simulink model "sim_kalman"  (R2024b)
settings: Solver=ode4  StartTime=t_0  StopTime=t_f  FixedStep=dt  RelTol=1e-8
libraries: simulink x1
settings Model: SimulationMode=accelerator  Creator=yevge  LastModifiedBy=Aiden Gaydos
settings DebuggingCC: AlgebraicLoopMsg=error  CheckMatrixSingularityMsg=error

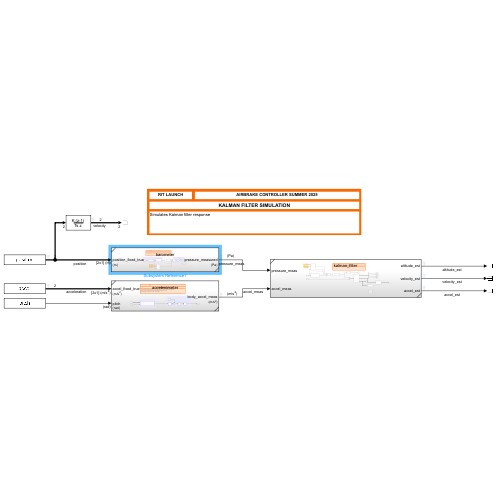
[thumbnail: Simulink's stored preview of the top-level diagram]
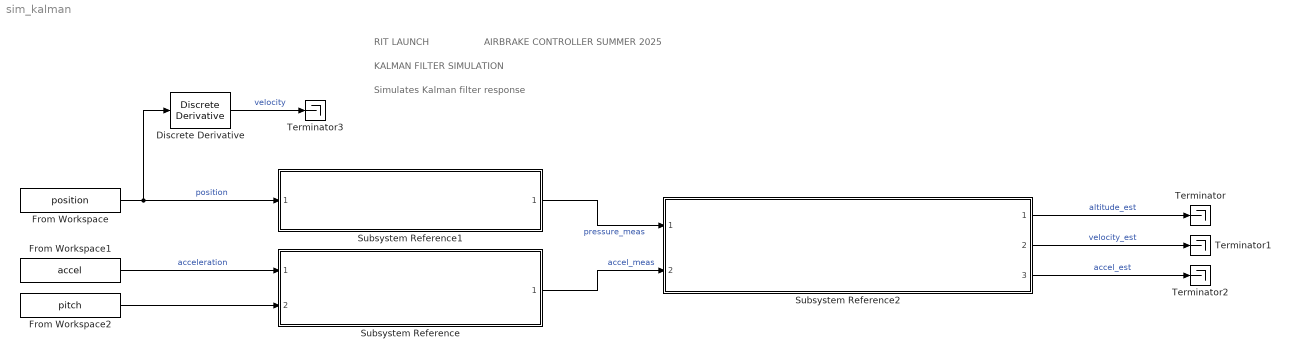
== system sim_kalman ==
  note: AIRBRAKE CONTROLLER SUMMER 2025
  note: RIT LAUNCH
  note: KALMAN FILTER SIMULATION
  note: Simulates Kalman filter response
  Discrete Derivative : simulink/Discrete/Discrete Derivative  gainval=1  ICPrevScaledInput=0.0  OutMin=[]  OutMax=[]  OutDataType=fixdt(1, 16)  OutScaling=2^-10  DoSatur=off
  From Workspace : FromWorkspace  VariableName=position
  From Workspace1 : FromWorkspace  VariableName=accel
  From Workspace2 : FromWorkspace  VariableName=pitch
  Subsystem Reference : Subsystem  ReferencedSubsystem=accelerometer
  Subsystem Reference1 : Subsystem  ReferencedSubsystem=barometer
  Subsystem Reference2 : Subsystem  ReferencedSubsystem=kalman_filter
  Terminator{,1..3} (4 alike) : Terminator
  wires:
  From Workspace/1 -> Discrete Derivative/1, Subsystem Reference1/1  "position"
  From Workspace1/1 -> Subsystem Reference/1  "acceleration"
  From Workspace2/1 -> Subsystem Reference/2
  Subsystem Reference/1 -> Subsystem Reference2/2  "accel_meas"
  Subsystem Reference1/1 -> Subsystem Reference2/1  "pressure_meas"
  Subsystem Reference2/1 -> Terminator/1  "altitude_est"
  Subsystem Reference2/2 -> Terminator1/1  "velocity_est"
  Subsystem Reference2/3 -> Terminator2/1  "accel_est"
  Discrete Derivative/1 -> Terminator3/1  "velocity"
